simulink model "motorModel"  (R2015a)
settings: Solver=ode45  StartTime=0.0  StopTime=1  RelTol=1e-3
values from neighbouring files (symbols this model uses):
  b = 0.000232    [motorModel.mat]
  Grr = 9.54929659643    [motorModel.mat]
  Gs = 1    [motorModel.mat]
  Gt = 0.014    [motorModel.mat]
  J = 2.50210296e-05    [motorModel.mat]
  Ke = 0.1    [motorModel.mat]
  Kt = 0.1    [motorModel.mat]
  L = 0.00527    [motorModel.mat]
  R = 4    [motorModel.mat]
settings Model: Creator=tabdallah1518  LastModifiedBy=tabdallah1518

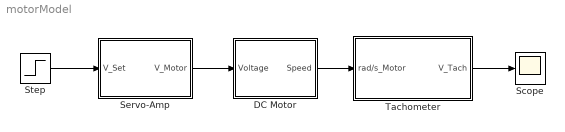
== system motorModel ==
  DC Motor : Subsystem
  Scope : Scope
  Servo-Amp : Subsystem
  Step : Step  Time=0  After=10  SampleTime=0
  Tachometer : Subsystem
  wires:
  DC Motor/1(Speed) -> Tachometer/1(rad/s_Motor)
  Step/1 -> Servo-Amp/1(V_Set)
  Servo-Amp/1(V_Motor) -> DC Motor/1(Voltage)
  Tachometer/1("V_Tach ") -> Scope/1

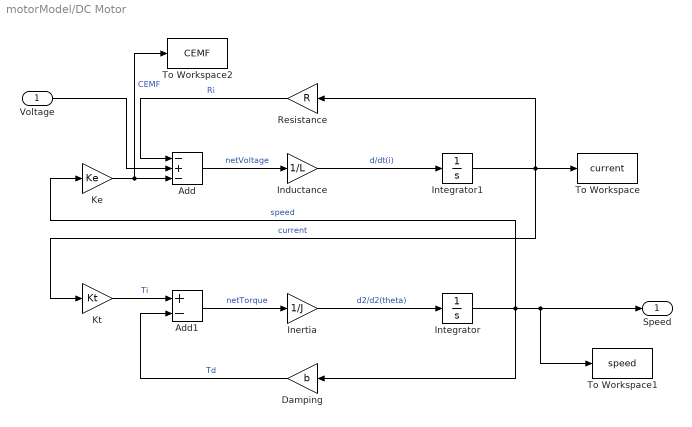
== system motorModel/DC Motor ==
  Voltage : Inport
  Add : Sum  Inputs=-+-
  Add1 : Sum  Inputs=+-
  Damping : Gain  Gain=b
  Inductance : Gain  Gain=1/L
  Inertia : Gain  Gain=1/J
  Integrator : Integrator
  Integrator1 : Integrator
  Ke : Gain  Gain=Ke
  Kt : Gain  Gain=Kt
  Resistance : Gain  Gain=R
  To Workspace : ToWorkspace  VariableName=current  SaveFormat=Timeseries  SampleTime=-1
  To Workspace1 : ToWorkspace  VariableName=speed  SaveFormat=Timeseries  SampleTime=-1
  To Workspace2 : ToWorkspace  VariableName=CEMF  SaveFormat=Timeseries  SampleTime=-1
  Speed : Outport
  wires:
  Add1/1 -> Inertia/1  "netTorque"
  Inertia/1 -> Integrator/1  "d2/d2(theta)"
  Integrator1/1 -> To Workspace/1, Resistance/1, Kt/1  "current"
  Integrator/1 -> To Workspace1/1, Speed/1, Ke/1, Damping/1  "speed"
  Inductance/1 -> Integrator1/1  "d/dt(i)"
  Add/1 -> Inductance/1  "netVoltage"
  Damping/1 -> Add1/2  "Td"
  Resistance/1 -> Add/1  "Ri"
  Kt/1 -> Add1/1  "Ti"
  Ke/1 -> To Workspace2/1, Add/3  "CEMF"
  Voltage/1 -> Add/2

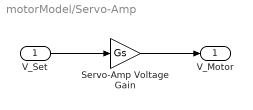
== system motorModel/Servo-Amp ==
  V_Set : Inport
  Servo-Amp Voltage Gain : Gain  Gain=Gs
  V_Motor : Outport
  wires:
  V_Set/1 -> Servo-Amp Voltage Gain/1
  Servo-Amp Voltage Gain/1 -> V_Motor/1

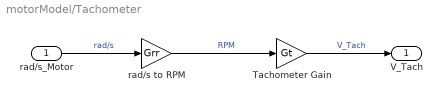
== system motorModel/Tachometer ==
  rad/s_Motor : Inport
  Tachometer Gain : Gain  Gain=Gt
  rad/s to RPM : Gain  Gain=Grr
  "V_Tach " : Outport
  wires:
  rad/s_Motor/1 -> rad/s to RPM/1  "rad/s"
  Tachometer Gain/1 -> "V_Tach "/1  "V_Tach"
  rad/s to RPM/1 -> Tachometer Gain/1  "RPM"
